simulink model "QuadOLSimR2017b"  (Simulink 9.0)
settings: Solver=ode45  StartTime=0.0  StopTime=500  MaxStep=0.01  RelTol=1e-3  EnableMultiTasking=on
values from neighbouring files (symbols this model uses):
  g = 9.81    [hw04_QuadOLPlots.m]    (also in hw04_QuadPlots.m)
  h0 = 0    [hw04_QuadOLPlots.m]    (also in hw04_QuadPlots.m)
  hbar = 1    [hw04_QuadOLPlots.m]
  hdot0 = 0    [hw04_QuadOLPlots.m]    (also in hw04_QuadPlots.m)
  kT = 5.276e-4    (= 0.0005276)    [hw04_QuadOLPlots.m]    (also in hw04_QuadPlots.m)
  m = 65e-3    (= 0.065)    [hw04_QuadOLPlots.m]    (also in hw04_QuadPlots.m)
  umax = 500    [hw04_QuadOLPlots.m]    (also in hw04_QuadPlots.m)
  umin = 0    [hw04_QuadOLPlots.m]    (also in hw04_QuadPlots.m)
settings Model: Creator=pjseiler  LastModifiedBy=pjseiler
settings DataIOCC: LimitDataPoints=on  SignalLoggingSaveFormat=ModelDataLogs
settings OptimizationCC: ExpressionDepthLimit=2147483647
settings DebuggingCC: SolverPrmCheckMsg=warning  FcnCallInpInsideContextMsg=warning  StateNameClashWarn=warning  SFExecutionAtInitializationDiag=warning
settings GRTTargetCC: GeneratePreprocessorConditionals=Disable all  CombineOutputUpdateFcns=off  GRTInterface=on

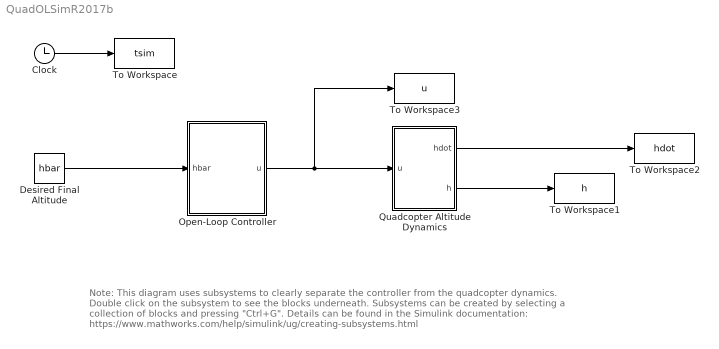
== system QuadOLSimR2017b ==
  note: Note: This diagram uses subsystems to clearly separate the controller from the quadcopter dynamics.
      | Double click on the subsystem to see the blocks underneath. Subsystems can be created by selecting
      | a collection of blocks and pressing "Ctrl+G". Details can be found in the Simulink documentation:
      | https://www.mathworks.com/help/simulink/ug/creating-subsystems.html
  Clock : Clock
  Desired Final Altitude : Constant  Value=hbar
  Open-Loop Controller : Subsystem
  Quadcopter Altitude Dynamics : Subsystem
  To Workspace : ToWorkspace  VariableName=tsim  SampleTime=-1
  To Workspace1 : ToWorkspace  VariableName=h  SampleTime=-1
  To Workspace2 : ToWorkspace  VariableName=hdot  SampleTime=-1
  To Workspace3 : ToWorkspace  VariableName=u  SampleTime=-1
  wires:
  Clock/1 -> To Workspace/1
  Quadcopter Altitude Dynamics/1(hdot) -> To Workspace2/1
  Quadcopter Altitude Dynamics/2(h) -> To Workspace1/1
  Desired Final Altitude/1 -> Open-Loop Controller/1(hbar)
  Open-Loop Controller/1(u) -> To Workspace3/1, Quadcopter Altitude Dynamics/1(u)

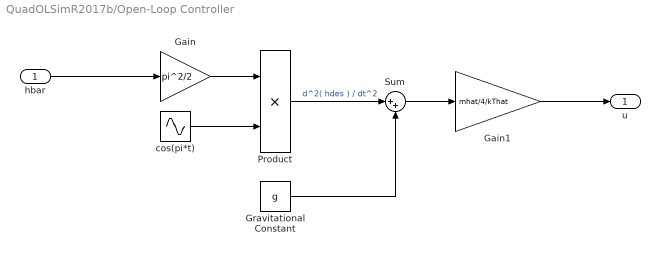
== system QuadOLSimR2017b/Open-Loop Controller ==
  hbar : Inport
  Gain : Gain  Gain=pi^2/2
  Gain1 : Gain  Gain=mhat/4/kThat
  Gravitational Constant : Constant  Value=g
  Product : Product
  Sum : Sum  Inputs=|++
  cos(pi*t) : Sin  Frequency=pi  Phase=pi/2  SampleTime=0
  u : Outport
  wires:
  Product/1 -> Sum/1  "d^2( hdes ) / dt^2"
  cos(pi*t)/1 -> Product/2
  Sum/1 -> Gain1/1
  Gain1/1 -> u/1
  Gravitational Constant/1 -> Sum/2
  hbar/1 -> Gain/1
  Gain/1 -> Product/1

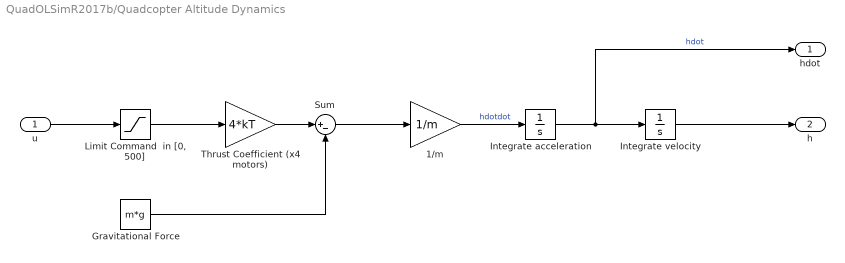
== system QuadOLSimR2017b/Quadcopter Altitude Dynamics ==
  u : Inport
  1/m : Gain  Gain=1/m
  Gravitational Force : Constant  Value=m*g
  Integrate acceleration : Integrator  InitialCondition=hdot0
  Integrate velocity : Integrator  InitialCondition=h0
  "Limit Command  in [0, 500]" : Saturate  UpperLimit=umax  LowerLimit=umin
  Sum : Sum  Inputs=|+-
  Thrust Coefficient (x4 motors) : Gain  Gain=4*kT
  hdot : Outport
  h : Outport  Port=2
  wires:
  Integrate acceleration/1 -> hdot/1, Integrate velocity/1  "hdot"
  Sum/1 -> 1/m/1
  Thrust Coefficient (x4 motors)/1 -> Sum/1
  u/1 -> "Limit Command  in [0, 500]"/1
  "Limit Command  in [0, 500]"/1 -> Thrust Coefficient (x4 motors)/1
  1/m/1 -> Integrate acceleration/1  "hdotdot"
  Gravitational Force/1 -> Sum/2
  Integrate velocity/1 -> h/1
